simulink model "IA331_Rubtsov_Lab11"  (R2023b)
settings: Solver=VariableStepAuto  StartTime=0.0  StopTime=1000  RelTol=1e-3
model workspace (MAT data in the model file):
  lambda = 0.2
  mu = 1
values from neighbouring files (symbols this model uses):
  m = 200    [IA331_Rubtsov_Lab1_3.m]    (also in IA331_Rubtsov_Lab4.m = 10; IA331_Rubtsov_Lab5.m = 1)
  n = length(x)    [IA331_Rubtsov_Lab2.m]    (also in IA331_Rubtsov_Lab3_2.m = sample_points(i); IA331_Rubtsov_Lab3_3.m = n_vals(i); IA331_Rubtsov_Lab4.m = 10)
settings Model: Creator=error  LastModifiedBy=error

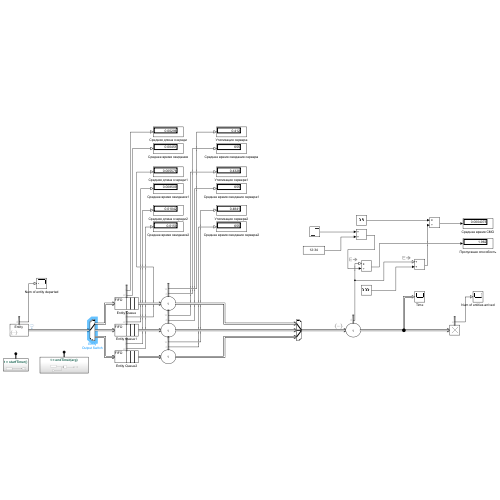
[thumbnail: Simulink's stored preview of the top-level diagram]
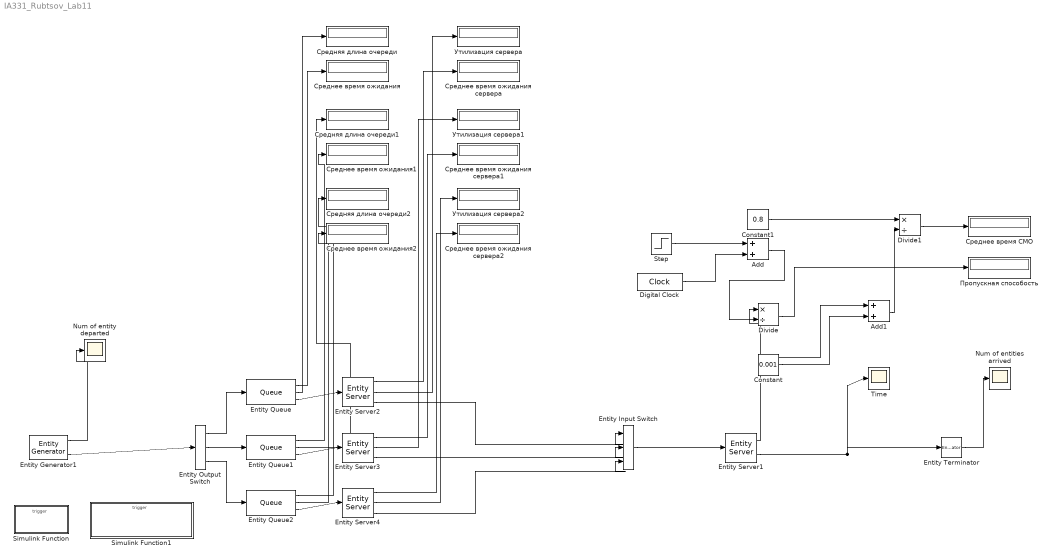
== system IA331_Rubtsov_Lab11 ==
  Add : Sum
  Add1 : Sum
  Constant : Constant  Value=0.001
  Constant1 : Constant  Value=0.8
  Digital Clock : DigitalClock
  Divide : Product  Inputs=*/
  Divide1 : Product  Inputs=*/
  Entity Input Switch : EntityInputSwitch  InputPortMessageModes=m,m,m  OutputPortMessageModes=m  NumberInputPorts=3
      settings: InputPortMap=u1,u2,u3
  Entity Output Switch : EntityOutputSwitch  InputPortMessageModes=m  OutputPortMessageModes=m,m,m  NumberOutputPorts=3  SwitchingCriterion=Round robin  SwitchAttributeName=Attribute1
      settings: OutputPortMap=o0,o1,o2
  Entity Generator1 : EntityGenerator  OutputPortMessageModes=n,m  TimeSource=MATLAB action  IntergenerationTimeAction=|  GenerateAction=entity.arrivalTime = startTimer();  AttributeName=ServiceTime|arrivalTime|time  AttributeInitialValue=exprnd(1/mu)|0|0  NumberEntitiesDeparted=on  EntityType=Structured  EntityTypeName=Entity
      | persistent rngInit;
      | if isempty(rngInit)
      |     rng(12345);
      |     rngInit = true;
      | end
      | 
      | dt = rand(1, 1);
      | 
      | x = -lambda * log(1 - rand());
      settings: OutputPortMap=o0,o3
  Entity Queue : Queue  InputPortMessageModes=m  OutputPortMessageModes=n,n,m  AverageWait=on  AverageQueueLength=on
      settings: OutputPortMap=o2,o3,o5
  Entity Queue1 : Queue  InputPortMessageModes=m  OutputPortMessageModes=n,n,m  AverageWait=on  AverageQueueLength=on
      settings: OutputPortMap=o2,o3,o5
  Entity Queue2 : Queue  InputPortMessageModes=m  OutputPortMessageModes=n,n,m  AverageWait=on  AverageQueueLength=on
      settings: OutputPortMap=o2,o3,o5
  Entity Server1 : EntityServer  InputPortMessageModes=m  OutputPortMessageModes=n,m  Capacity=1  ServiceTimeSource=Attribute  EntryAction=entity.time = endTimer(entity.arrivalTime);  NumberEntitiesDeparted=on
      settings: OutputPortMap=o0,o9
  Entity Server2 : EntityServer  InputPortMessageModes=m  OutputPortMessageModes=n,n,m  Capacity=1  ServiceTimeSource=Attribute  NumberEntitiesDeparted=on  AverageWait=on
      settings: OutputPortMap=o0,o4,o9
  Entity Server3 : EntityServer  InputPortMessageModes=m  OutputPortMessageModes=n,n,m  Capacity=1  ServiceTimeSource=Attribute  NumberEntitiesDeparted=on  AverageWait=on
      settings: OutputPortMap=o0,o4,o9
  Entity Server4 : EntityServer  InputPortMessageModes=m  OutputPortMessageModes=n,n,m  Capacity=1  ServiceTimeSource=Attribute  NumberEntitiesDeparted=on  AverageWait=on
      settings: OutputPortMap=o0,o4,o9
  Entity Terminator : EntityTerminator  InputPortMessageModes=m  NumberEntitiesArrived=on
      settings: OutputPortMap=o0
  Num of entities arrived : Scope
  Num of entity departed : Scope
  Simulink Function : Subsystem  TreatAsAtomicUnit=on
  Simulink Function1 : Subsystem  TreatAsAtomicUnit=on
  Step : Step  SampleTime=0
  Time : Scope
  Пропускная способость : Display
  Среднее время СМО : Display
  Среднее время ожидания : Display
  Среднее время ожидания сервера : Display
  Среднее время ожидания сервера1 : Display
  Среднее время ожидания сервера2 : Display
  Среднее время ожидания1 : Display
  Среднее время ожидания2 : Display
  Средняя длина очереди : Display
  Средняя длина очереди1 : Display
  Средняя длина очереди2 : Display
  Утилизация сервера : Display
  Утилизация сервера1 : Display
  Утилизация сервера2 : Display
  wires:
  Entity Generator1/1 -> Num of entity departed/1
  Entity Generator1/2 -> Entity Output Switch/1
  Entity Server1/2 -> Time/1, Entity Terminator/1
  Entity Server1/1 -> Add1/1, Divide/1
  Constant/1 -> Add1/2
  Step/1 -> Add/1
  Digital Clock/1 -> Add/2
  Add/1 -> Divide/2
  Divide/1 -> Пропускная способость/1
  Add1/1 -> Divide1/2
  Divide1/1 -> Среднее время СМО/1
  Entity Terminator/1 -> Num of entities arrived/1
  Constant1/1 -> Divide1/1
  Entity Output Switch/1 -> Entity Queue/1
  Entity Output Switch/2 -> Entity Queue1/1
  Entity Output Switch/3 -> Entity Queue2/1
  Entity Queue/3 -> Entity Server2/1
  Entity Queue1/3 -> Entity Server3/1
  Entity Queue2/3 -> Entity Server4/1
  Entity Server2/3 -> Entity Input Switch/1
  Entity Server3/3 -> Entity Input Switch/2
  Entity Server4/3 -> Entity Input Switch/3
  Entity Queue/2 -> Средняя длина очереди/1
  Entity Queue/1 -> Среднее время ожидания/1
  Entity Queue1/2 -> Средняя длина очереди1/1
  Entity Queue1/1 -> Среднее время ожидания1/1
  Entity Queue2/2 -> Средняя длина очереди2/1
  Entity Queue2/1 -> Среднее время ожидания2/1
  Entity Server2/2 -> Утилизация сервера/1
  Entity Server2/1 -> Среднее время ожидания сервера/1
  Entity Server3/2 -> Утилизация сервера1/1
  Entity Server3/1 -> Среднее время ожидания сервера1/1
  Entity Server4/2 -> Утилизация сервера2/1
  Entity Server4/1 -> Среднее время ожидания сервера2/1
  Entity Input Switch/1 -> Entity Server1/1

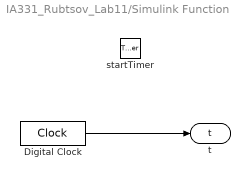
== system IA331_Rubtsov_Lab11/Simulink Function ==
  startTimer : TriggerPort  TriggerType=function-call  IsSimulinkFunction=on  FunctionName=startTimer  FunctionVisibility=scoped  VariantControl=(inherit)
  Digital Clock : DigitalClock  SampleTime=-1
  t : ArgOut  DisableCoverage=on  ArgumentName=t
  wires:
  Digital Clock/1 -> t/1

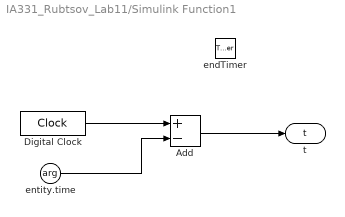
== system IA331_Rubtsov_Lab11/Simulink Function1 ==
  endTimer : TriggerPort  TriggerType=function-call  IsSimulinkFunction=on  FunctionName=endTimer  FunctionVisibility=scoped  VariantControl=(inherit)
  Add : Sum  Inputs=+-
  Digital Clock : DigitalClock  SampleTime=-1
  entity.time : ArgIn  ArgumentName=arg
  t : ArgOut  DisableCoverage=on  ArgumentName=t
  wires:
  Digital Clock/1 -> Add/1
  entity.time/1 -> Add/2
  Add/1 -> t/1
